simulink model "flexpes_phctrlr_sys"  (R2025b)
settings: Solver=VariableStepAuto  StartTime=0.0  StopTime=1e-6  RelTol=1e-3
values from neighbouring files (symbols this model uses):
  debouncer_cycles = 5    [choPLL_loop_impl.m]
  F_lock_thr = 1    [choPLL_loop_impl.m]
  FPGA_CLK = 125e6    (= 125000000)    [choPLL_loop_impl.m]
  FPGA_Ts = 1./FPGA_CLK    (= 8e-09)    [choPLL_loop_impl.m]
  IIR_C_X = G_loopfilt*my_num_loop_filtZ(1)    [choPLL_loop_impl.m]
  IIR_C_X1 = G_loopfilt*my_num_loop_filtZ(2)    [choPLL_loop_impl.m]
  IIR_C_Y1 = -my_den_loop_filtZ(2)    [choPLL_loop_impl.m]
  max_unwrap_periods = 50    [choPLL_loop_impl.m]
  PFD_CLK = 100e3    (= 100000)    [choPLL_loop_impl.m]
  PFD_Ts = 1./PFD_CLK    (= 1e-05)    [choPLL_loop_impl.m]
  PH_lock_thr = 4    [choPLL_loop_impl.m]
  PHCTRLR_CLK = 100    [choPLL_loop_impl.m]
  PHCTRLR_Ts = 1./PHCTRLR_CLK    (= 0.01)    [choPLL_loop_impl.m]
  TDC_cnt_per_period = round(FPGA_CLK/Fref)    [choPLL_loop_impl.m]
  unwrap_res_period_thr = 0    [choPLL_loop_impl.m]
  unwrap_reset_inhibit_cycles = 20000    [choPLL_loop_impl.m]
  wrap_detect_thr = round(TDC_cnt_per_period*0.55)    [choPLL_loop_impl.m]
libraries: hdlBasic x276, hdlUtilities x4, hdlDSPIP x4, vmcUtilities x1
(part 2 of 3)

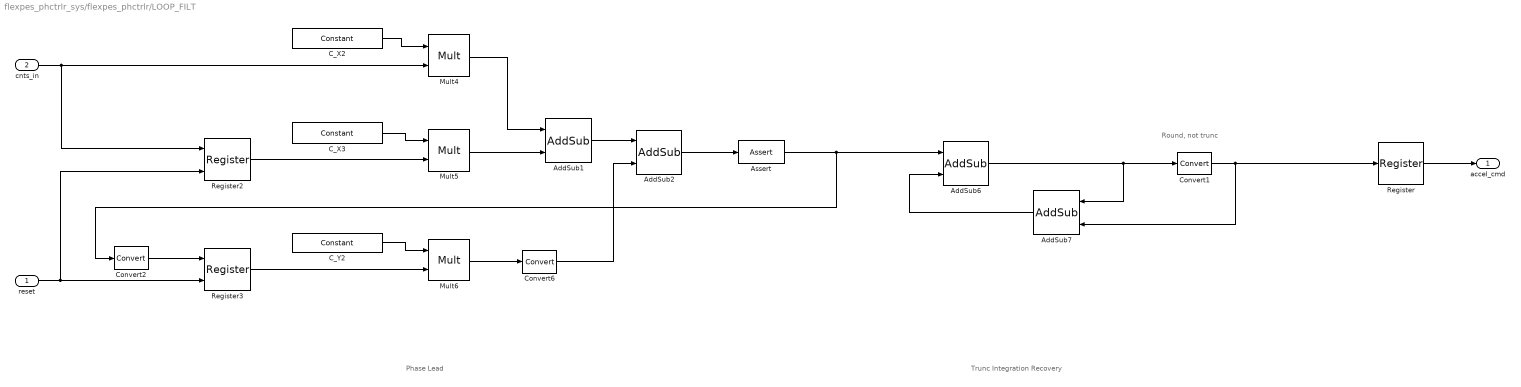
== system flexpes_phctrlr_sys/flexpes_phctrlr/LOOP_FILT ==
  note: Round, not trunc
  note: Phase Lead
  note: Trunc Integration Recovery
  reset : Inport
  cnts_in : Inport  Port=2
  AddSub1 : hdlBasic/AddSub  mode=Addition  use_carryin=off  use_carryout=off  en=off  latency=0  precision=Full  arith_type=Unsigned  n_bits=16  bin_pt=14  quantization=Truncate  overflow=Wrap  use_behavioral_HDL=off  hw_selection=Fabric  pipelined=off  XmcBlockStatus=1  maskContainerNames=tabcontainer1  block_type=addsub  block_config=sysgen:Addsub_config
  AddSub2 : hdlBasic/AddSub  mode=Addition  use_carryin=off  use_carryout=off  en=off  latency=0  precision=Full  arith_type=Unsigned  n_bits=16  bin_pt=14  quantization=Truncate  overflow=Wrap  use_behavioral_HDL=off  hw_selection=Fabric  pipelined=off  XmcBlockStatus=1  maskContainerNames=tabcontainer1  block_type=addsub  block_config=sysgen:Addsub_config
  AddSub6 : hdlBasic/AddSub  mode=Addition  use_carryin=off  use_carryout=off  en=off  latency=0  precision=User Defined  arith_type="Signed  (2's comp)"  n_bits=44  bin_pt=24  quantization="Round  (unbiased: +/- Inf)"  overflow=Saturate  use_behavioral_HDL=off  hw_selection=Fabric  pipelined=off  XmcBlockStatus=1  maskContainerNames=tabcontainer1  block_type=addsub  block_config=sysgen:Addsub_config
  AddSub7 : hdlBasic/AddSub  mode=Subtraction  use_carryin=off  use_carryout=off  en=off  latency=1  precision=User Defined  arith_type="Signed  (2's comp)"  n_bits=44  bin_pt=24  quantization="Round  (unbiased: +/- Inf)"  overflow=Saturate  use_behavioral_HDL=off  hw_selection=Fabric  pipelined=off  XmcBlockStatus=1  maskContainerNames=tabcontainer1  block_type=addsub  block_config=sysgen:Addsub_config
  Assert : hdlBasic/Assert  assert_type=off  type_source=Explicitly  gui_display_data_type=Fixed-point  arith_type=Signed (2's comp)  n_bits=16  bin_pt=14  preci_type=Single  exp_width=8  frac_width=24  assert_rate=on  rate_source=Explicitly  period=PHCTRLR_Ts  output_port=on  XmcBlockStatus=1  maskContainerNames=group1  block_type=assert  block_config=sysgen:assert_config  block_width=609  block_height=900
  C_X2 : hdlBasic/Constant  const=IIR_C_X  gui_display_data_type=Fixed-point  arith_type=Signed (2's comp)  n_bits=18  bin_pt=17  preci_type=Single  exp_width=8  frac_width=24  explicit_period=on  period=PHCTRLR_Ts  XmcBlockStatus=1  maskContainerNames=tabcontainer1  block_type=constant  block_config=sysgen:Constant_config
  C_X3 : hdlBasic/Constant  const=IIR_C_X1  gui_display_data_type=Fixed-point  arith_type=Signed (2's comp)  n_bits=18  bin_pt=17  preci_type=Single  exp_width=8  frac_width=24  explicit_period=on  period=PHCTRLR_Ts  XmcBlockStatus=1  maskContainerNames=tabcontainer1  block_type=constant  block_config=sysgen:Constant_config
  C_Y2 : hdlBasic/Constant  const=IIR_C_Y1  gui_display_data_type=Fixed-point  arith_type=Signed (2's comp)  n_bits=18  bin_pt=17  preci_type=Single  exp_width=8  frac_width=24  explicit_period=on  period=PHCTRLR_Ts  XmcBlockStatus=1  maskContainerNames=tabcontainer1  block_type=constant  block_config=sysgen:Constant_config
  Convert1 : hdlBasic/Convert  gui_display_data_type=Fixed-point  arith_type=Signed (2's comp)  n_bits=22  bin_pt=0  float_type=Single  exp_bits=8  fraction_bits=24  quantization="Round  (unbiased: Even Values)"  overflow=Saturate  en=off  latency=0  pipeline=off  XmcBlockStatus=1  maskContainerNames=group2  block_type=convert  block_config=sysgen:Convert_config  block_width=595  block_height=885
  Convert2 : hdlBasic/Convert  gui_display_data_type=Fixed-point  arith_type=Signed (2's comp)  n_bits=42  bin_pt=24  float_type=Single  exp_bits=8  fraction_bits=24  quantization="Round  (unbiased: Even Values)"  overflow=Saturate  en=off  latency=0  pipeline=off  XmcBlockStatus=1  maskContainerNames=group2  block_type=convert  block_config=sysgen:Convert_config  block_width=595  block_height=885
  Convert6 : hdlBasic/Convert  gui_display_data_type=Fixed-point  arith_type=Signed (2's comp)  n_bits=43  bin_pt=24  float_type=Single  exp_bits=8  fraction_bits=24  quantization="Round  (unbiased: Even Values)"  overflow=Saturate  en=off  latency=0  pipeline=off  XmcBlockStatus=1  maskContainerNames=group2  block_type=convert  block_config=sysgen:Convert_config  block_width=595  block_height=885
  Mult4 : hdlBasic/Mult  precision=Full  arith_type="Signed  (2's comp)"  n_bits=16  bin_pt=14  quantization=Truncate  overflow=Wrap  en=off  latency=0  opt_float=off  fp_mult_usage=No Usage  use_behavioral_HDL=off  opt=Speed  use_embedded=on  optimum_pipeline=off  pipeline=on  use_rpm=on  placement_style=Triangular  XmcBlockStatus=1  maskContainerNames=group1  block_type=mult  block_config=sysgen:Mult_config  block_width=598  block_height=876
  Mult5 : hdlBasic/Mult  precision=Full  arith_type="Signed  (2's comp)"  n_bits=16  bin_pt=14  quantization=Truncate  overflow=Wrap  en=off  latency=0  opt_float=off  fp_mult_usage=No Usage  use_behavioral_HDL=off  opt=Speed  use_embedded=on  optimum_pipeline=off  pipeline=on  use_rpm=on  placement_style=Triangular  XmcBlockStatus=1  maskContainerNames=group1  block_type=mult  block_config=sysgen:Mult_config  block_width=598  block_height=876
  Mult6 : hdlBasic/Mult  precision=Full  arith_type="Signed  (2's comp)"  n_bits=16  bin_pt=14  quantization=Truncate  overflow=Wrap  en=off  latency=0  opt_float=off  fp_mult_usage=No Usage  use_behavioral_HDL=off  opt=Speed  use_embedded=on  optimum_pipeline=off  pipeline=on  use_rpm=on  placement_style=Triangular  XmcBlockStatus=1  maskContainerNames=group1  block_type=mult  block_config=sysgen:Mult_config  block_width=598  block_height=876
  Register : hdlBasic/Register  init=0  rst=off  en=off  XmcBlockStatus=1  maskContainerNames=tabcontainer1  block_type=register  block_config=sysgen:Register_config
  Register2 : hdlBasic/Register  init=0  rst=on  en=off  XmcBlockStatus=1  maskContainerNames=tabcontainer1  block_type=register  block_config=sysgen:Register_config
  Register3 : hdlBasic/Register  init=0  rst=on  en=off  XmcBlockStatus=1  maskContainerNames=tabcontainer1  block_type=register  block_config=sysgen:Register_config
  accel_cmd : Outport
  wires:
  reset/1 -> Register2/2, Register3/2
  Convert6/1 -> AddSub2/2
  Mult4/1 -> AddSub1/1
  C_X3/1 -> Mult5/1
  Convert2/1 -> Register3/1
  Mult5/1 -> AddSub1/2
  C_X2/1 -> Mult4/1
  Mult6/1 -> Convert6/1
  cnts_in/1 -> Mult4/2, Register2/1
  Register2/1 -> Mult5/2
  C_Y2/1 -> Mult6/1
  AddSub2/1 -> Assert/1
  AddSub1/1 -> AddSub2/1
  Register3/1 -> Mult6/2
  Register/1 -> accel_cmd/1
  AddSub6/1 -> AddSub7/1, Convert1/1
  Convert1/1 -> Register/1, AddSub7/2
  AddSub7/1 -> AddSub6/2
  Assert/1 -> Convert2/1, AddSub6/1

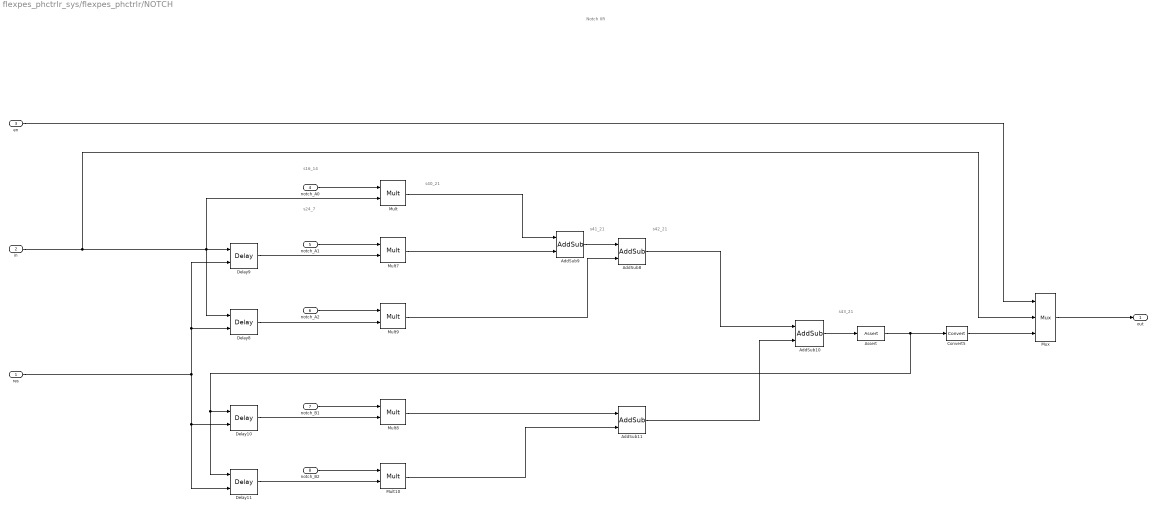
== system flexpes_phctrlr_sys/flexpes_phctrlr/NOTCH ==
  note: s16_14
  note: Notch IIR
  note: s24_7
  note: s40_21
  note: s42_21
  note: s43_21
  note: s41_21
  res : Inport
  in : Inport  Port=2
  en : Inport  Port=3
  notch_A0 : Inport  Port=4  OutDataTypeStr=fixdt(1,16,14)
  notch_A1 : Inport  Port=5  OutDataTypeStr=fixdt(1,16,14)
  notch_A2 : Inport  Port=6  OutDataTypeStr=fixdt(1,16,14)
  notch_B1 : Inport  Port=7  OutDataTypeStr=fixdt(1,16,14)
  notch_B2 : Inport  Port=8  OutDataTypeStr=fixdt(1,16,14)
  AddSub10 : hdlBasic/AddSub  mode=Subtraction  use_carryin=off  use_carryout=off  en=off  latency=0  precision=Full  arith_type="Signed  (2's comp)"  n_bits=62  bin_pt=40  quantization="Round  (unbiased: +/- Inf)"  overflow=Saturate  use_behavioral_HDL=off  hw_selection=Fabric  pipelined=off  XmcBlockStatus=1  maskContainerNames=tabcontainer1  block_type=addsub  block_config=sysgen:Addsub_config
  AddSub11 : hdlBasic/AddSub  mode=Addition  use_carryin=off  use_carryout=off  en=off  latency=0  precision=Full  arith_type="Signed  (2's comp)"  n_bits=62  bin_pt=40  quantization="Round  (unbiased: +/- Inf)"  overflow=Saturate  use_behavioral_HDL=off  hw_selection=Fabric  pipelined=off  XmcBlockStatus=1  maskContainerNames=tabcontainer1  block_type=addsub  block_config=sysgen:Addsub_config
  AddSub8 : hdlBasic/AddSub  mode=Addition  use_carryin=off  use_carryout=off  en=off  latency=0  precision=Full  arith_type=Unsigned  n_bits=16  bin_pt=14  quantization=Truncate  overflow=Wrap  use_behavioral_HDL=off  hw_selection=Fabric  pipelined=off  XmcBlockStatus=1  maskContainerNames=tabcontainer1  block_type=addsub  block_config=sysgen:Addsub_config
  AddSub9 : hdlBasic/AddSub  mode=Addition  use_carryin=off  use_carryout=off  en=off  latency=0  precision=Full  arith_type=Unsigned  n_bits=16  bin_pt=14  quantization=Truncate  overflow=Wrap  use_behavioral_HDL=off  hw_selection=Fabric  pipelined=off  XmcBlockStatus=1  maskContainerNames=tabcontainer1  block_type=addsub  block_config=sysgen:Addsub_config
  Assert : hdlBasic/Assert  assert_type=off  type_source=Explicitly  gui_display_data_type=Fixed-point  arith_type=Signed (2's comp)  n_bits=16  bin_pt=14  preci_type=Single  exp_width=8  frac_width=24  assert_rate=on  rate_source=Explicitly  period=PHCTRLR_Ts  output_port=on  XmcBlockStatus=1  maskContainerNames=group1  block_type=assert  block_config=sysgen:assert_config  block_width=609  block_height=900
  Convert5 : hdlBasic/Convert  gui_display_data_type=Fixed-point  arith_type=Signed (2's comp)  n_bits=24  bin_pt=7  float_type=Single  exp_bits=8  fraction_bits=24  quantization="Round  (unbiased: Even Values)"  overflow=Saturate  en=off  latency=1  pipeline=off  XmcBlockStatus=1  maskContainerNames=group2  block_type=convert  block_config=sysgen:Convert_config  block_width=595  block_height=885
  Delay10 : hdlBasic/Delay  rst=on  en=off  latency=1  reg_retiming=off  XmcBlockStatus=1  maskContainerNames=group1  block_type=delay  block_config=sysgen:Delay_config
  Delay11 : hdlBasic/Delay  rst=on  en=off  latency=2  reg_retiming=off  XmcBlockStatus=1  maskContainerNames=group1  block_type=delay  block_config=sysgen:Delay_config
  Delay8 : hdlBasic/Delay  rst=on  en=off  latency=2  reg_retiming=off  XmcBlockStatus=1  maskContainerNames=group1  block_type=delay  block_config=sysgen:Delay_config
  Delay9 : hdlBasic/Delay  rst=on  en=off  latency=1  reg_retiming=off  XmcBlockStatus=1  maskContainerNames=group1  block_type=delay  block_config=sysgen:Delay_config
  Mult : hdlBasic/Mult  precision=Full  arith_type="Signed  (2's comp)"  n_bits=16  bin_pt=14  quantization=Truncate  overflow=Wrap  en=off  latency=0  opt_float=off  fp_mult_usage=No Usage  use_behavioral_HDL=off  opt=Speed  use_embedded=on  optimum_pipeline=off  pipeline=on  use_rpm=on  placement_style=Triangular  XmcBlockStatus=1  maskContainerNames=group1  block_type=mult  block_config=sysgen:Mult_config  block_width=598  block_height=876
  Mult10 : hdlBasic/Mult  precision=User Defined  arith_type="Signed  (2's comp)"  n_bits=41  bin_pt=21  quantization="Round  (unbiased: +/- Inf)"  overflow=Saturate  en=off  latency=0  opt_float=off  fp_mult_usage=No Usage  use_behavioral_HDL=off  opt=Speed  use_embedded=on  optimum_pipeline=off  pipeline=on  use_rpm=on  placement_style=Triangular  XmcBlockStatus=1  maskContainerNames=group1  block_type=mult  block_config=sysgen:Mult_config  block_width=598  block_height=876
  Mult7 : hdlBasic/Mult  precision=Full  arith_type="Signed  (2's comp)"  n_bits=16  bin_pt=14  quantization=Truncate  overflow=Wrap  en=off  latency=0  opt_float=off  fp_mult_usage=No Usage  use_behavioral_HDL=off  opt=Speed  use_embedded=on  optimum_pipeline=off  pipeline=on  use_rpm=on  placement_style=Triangular  XmcBlockStatus=1  maskContainerNames=group1  block_type=mult  block_config=sysgen:Mult_config  block_width=598  block_height=876
  Mult8 : hdlBasic/Mult  precision=User Defined  arith_type="Signed  (2's comp)"  n_bits=41  bin_pt=21  quantization="Round  (unbiased: +/- Inf)"  overflow=Saturate  en=off  latency=0  opt_float=off  fp_mult_usage=No Usage  use_behavioral_HDL=off  opt=Speed  use_embedded=on  optimum_pipeline=off  pipeline=on  use_rpm=on  placement_style=Triangular  XmcBlockStatus=1  maskContainerNames=group1  block_type=mult  block_config=sysgen:Mult_config  block_width=598  block_height=876
  Mult9 : hdlBasic/Mult  precision=Full  arith_type="Signed  (2's comp)"  n_bits=16  bin_pt=14  quantization=Truncate  overflow=Wrap  en=off  latency=0  opt_float=off  fp_mult_usage=No Usage  use_behavioral_HDL=off  opt=Speed  use_embedded=on  optimum_pipeline=off  pipeline=on  use_rpm=on  placement_style=Triangular  XmcBlockStatus=1  maskContainerNames=group1  block_type=mult  block_config=sysgen:Mult_config  block_width=598  block_height=876
  Mux : hdlBasic/Mux  inputs=2  en=off  latency=1  precision=Full  arith_type=Unsigned  n_bits=16  bin_pt=14  quantization=Truncate  overflow=Wrap  XmcBlockStatus=1  maskContainerNames=tabcontainer1  block_type=mux  block_config=sysgen:Mux_config
  out : Outport
  wires:
  AddSub11/1 -> AddSub10/2
  Mult7/1 -> AddSub9/2
  notch_A1/1 -> Mult7/1
  Mult9/1 -> AddSub8/2
  Delay9/1 -> Mult7/2
  in/1 -> Mux/2, Mult/2, Delay8/1, Delay9/1
  notch_B1/1 -> Mult8/1
  AddSub8/1 -> AddSub10/1
  Convert5/1 -> Mux/3
  AddSub10/1 -> Assert/1
  notch_A2/1 -> Mult9/1
  Delay8/1 -> Mult9/2
  notch_A0/1 -> Mult/1
  Mult10/1 -> AddSub11/2
  Mult8/1 -> AddSub11/1
  Delay10/1 -> Mult8/2
  Delay11/1 -> Mult10/2
  AddSub9/1 -> AddSub8/1
  en/1 -> Mux/1
  Mult/1 -> AddSub9/1
  res/1 -> Delay11/2, Delay10/2, Delay9/2, Delay8/2
  Mux/1 -> out/1
  notch_B2/1 -> Mult10/1
  Assert/1 -> Delay11/1, Delay10/1, Convert5/1

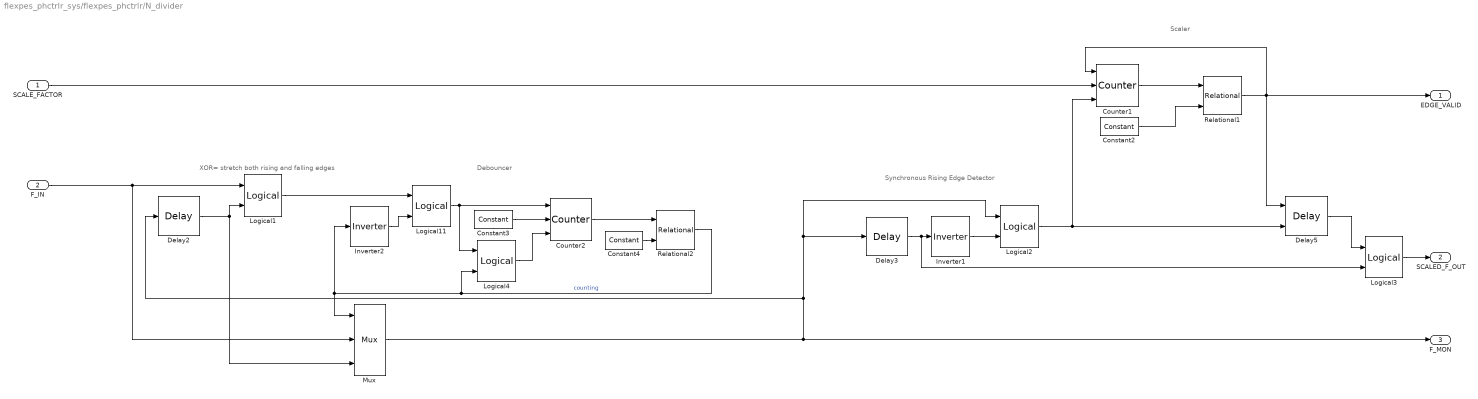
== system flexpes_phctrlr_sys/flexpes_phctrlr/N_divider ==
  note: XOR= stretch both rising and falling edges
  note: Debouncer
  note: Scaler
  note: Synchronous Rising Edge Detector
  SCALE_FACTOR : Inport
  F_IN : Inport  Port=2
  Constant2 : hdlBasic/Constant  const=1.0  gui_display_data_type=Fixed-point  arith_type=Unsigned  n_bits=16  bin_pt=0  preci_type=Single  exp_width=8  frac_width=24  explicit_period=off  period=1  XmcBlockStatus=1  maskContainerNames=tabcontainer1  block_type=constant  block_config=sysgen:Constant_config
  Constant3 : hdlBasic/Constant  const=debouncer_cycles  gui_display_data_type=Fixed-point  arith_type=Unsigned  n_bits=7  bin_pt=0  preci_type=Single  exp_width=8  frac_width=24  explicit_period=off  period=1  XmcBlockStatus=1  maskContainerNames=tabcontainer1  block_type=constant  block_config=sysgen:Constant_config
  Constant4 : hdlBasic/Constant  const=1  gui_display_data_type=Fixed-point  arith_type=Unsigned  n_bits=7  bin_pt=0  preci_type=Single  exp_width=8  frac_width=24  explicit_period=off  period=1  XmcBlockStatus=1  maskContainerNames=tabcontainer1  block_type=constant  block_config=sysgen:Constant_config
  Counter1 : hdlBasic/Counter  cnt_type=Free running  cnt_to=2  operation=Down  start_count=1  cnt_by_val=1  arith_type=Unsigned  n_bits=16  bin_pt=0  load_pin=on  rst=off  en=on  explicit_period=Explicit  period=FPGA_Ts  use_behavioral_HDL=off  implementation=Fabric  XmcBlockStatus=1  maskContainerNames=group1  block_type=counter  block_config=sysgen:Counter_config  block_width=531  block_height=1023
  Counter2 : hdlBasic/Counter  cnt_type=Free running  cnt_to=2  operation=Down  start_count=1  cnt_by_val=1  arith_type=Unsigned  n_bits=7  bin_pt=0  load_pin=on  rst=off  en=on  explicit_period=Explicit  period=FPGA_Ts  use_behavioral_HDL=off  implementation=Fabric  XmcBlockStatus=1  maskContainerNames=group1  block_type=counter  block_config=sysgen:Counter_config  block_width=531  block_height=1023
  Delay2 : hdlBasic/Delay  rst=off  en=off  latency=1  reg_retiming=off  XmcBlockStatus=1  maskContainerNames=group1  block_type=delay  block_config=sysgen:Delay_config
  Delay3 : hdlBasic/Delay  rst=off  en=off  latency=1  reg_retiming=off  XmcBlockStatus=1  maskContainerNames=group1  block_type=delay  block_config=sysgen:Delay_config
  Delay5 : hdlBasic/Delay  rst=off  en=on  latency=1  reg_retiming=off  XmcBlockStatus=1  maskContainerNames=group1  block_type=delay  block_config=sysgen:Delay_config
  Inverter1 : hdlBasic/Inverter  en=off  latency=0  XmcBlockStatus=1  maskContainerNames=group2  block_type=inv  block_config=sysgen:Inverter_config
  Inverter2 : hdlBasic/Inverter  en=off  latency=0  XmcBlockStatus=1  maskContainerNames=group2  block_type=inv  block_config=sysgen:Inverter_config
  Logical1 : hdlBasic/Logical  logical_function=XOR  inputs=2  en=off  latency=0  precision=Full  arith_type=Unsigned  n_bits=16  bin_pt=0  align_bp=on  overflow=[]  quantization=[]  XmcBlockStatus=1  maskContainerNames=tabcontainer1  block_type=logical  block_config=sysgen:Logical_config
  Logical11 : hdlBasic/Logical  logical_function=AND  inputs=2  en=off  latency=0  precision=Full  arith_type=Unsigned  n_bits=16  bin_pt=0  align_bp=on  overflow=[]  quantization=[]  XmcBlockStatus=1  maskContainerNames=tabcontainer1  block_type=logical  block_config=sysgen:Logical_config
  Logical2 : hdlBasic/Logical  logical_function=AND  inputs=2  en=off  latency=0  precision=Full  arith_type=Unsigned  n_bits=16  bin_pt=0  align_bp=on  overflow=[]  quantization=[]  XmcBlockStatus=1  maskContainerNames=tabcontainer1  block_type=logical  block_config=sysgen:Logical_config
  Logical3 : hdlBasic/Logical  logical_function=AND  inputs=2  en=off  latency=0  precision=Full  arith_type=Unsigned  n_bits=16  bin_pt=0  align_bp=on  overflow=[]  quantization=[]  XmcBlockStatus=1  maskContainerNames=tabcontainer1  block_type=logical  block_config=sysgen:Logical_config
  Logical4 : hdlBasic/Logical  logical_function=OR  inputs=2  en=off  latency=0  precision=Full  arith_type=Unsigned  n_bits=16  bin_pt=0  align_bp=on  overflow=[]  quantization=[]  XmcBlockStatus=1  maskContainerNames=tabcontainer1  block_type=logical  block_config=sysgen:Logical_config
  Mux : hdlBasic/Mux  inputs=2  en=off  latency=0  precision=Full  arith_type=Unsigned  n_bits=16  bin_pt=14  quantization=Truncate  overflow=Wrap  XmcBlockStatus=1  maskContainerNames=tabcontainer1  block_type=mux  block_config=sysgen:Mux_config
  Relational1 : hdlBasic/Relational  mode=a=b  op_type=Bool  en=off  latency=0  XmcBlockStatus=1  maskContainerNames=tabcontainer1  block_type=relational  block_config=sysgen:Relational_config
  Relational2 : hdlBasic/Relational  mode=a!=b  op_type=Bool  en=off  latency=0  XmcBlockStatus=1  maskContainerNames=tabcontainer1  block_type=relational  block_config=sysgen:Relational_config
  EDGE_VALID : Outport
  SCALED_F_OUT : Outport  Port=2
  F_MON : Outport  Port=3
  wires:
  Delay2/1 -> Logical1/2, Mux/3
  Logical2/1 -> Delay5/2, Counter1/3
  Constant4/1 -> Relational2/2
  Inverter2/1 -> Logical11/2
  Counter2/1 -> Relational2/1
  Constant3/1 -> Counter2/2
  Relational2/1 -> Mux/1, Inverter2/1, Logical4/2  "counting"
  Delay5/1 -> Logical3/1
  Delay3/1 -> Inverter1/1, Logical3/2
  F_IN/1 -> Logical1/1, Mux/2
  Counter1/1 -> Relational1/1
  Inverter1/1 -> Logical2/2
  Constant2/1 -> Relational1/2
  SCALE_FACTOR/1 -> Counter1/2
  Logical11/1 -> Logical4/1, Counter2/1
  Logical3/1 -> SCALED_F_OUT/1
  Logical4/1 -> Counter2/3
  Logical1/1 -> Logical11/1
  Relational1/1 -> EDGE_VALID/1, Delay5/1, Counter1/1
  Mux/1 -> F_MON/1, Delay2/1, Logical2/1, Delay3/1

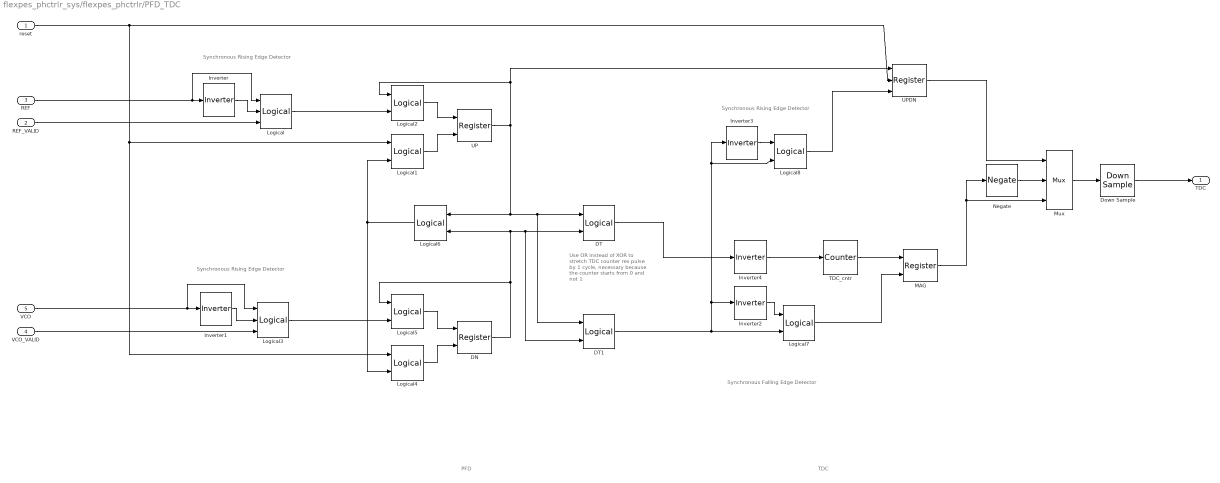
== system flexpes_phctrlr_sys/flexpes_phctrlr/PFD_TDC ==
  note: Synchronous Rising Edge Detector
  note: Synchronous Rising Edge Detector
  note: Synchronous Rising Edge Detector
  note: Synchronous Falling Edge Detector
  note: PFD
  note: TDC
  note: Use OR instead of XOR to
      | stretch TDC counter res
      | pulse by 1 cycle, necessary
      | because the counter starts
      | from 0 and not 1
  reset : Inport  SampleTime=FPGA_Ts
  REF_VALID : Inport  Port=2  SampleTime=FPGA_Ts
  REF : Inport  Port=3  SampleTime=FPGA_Ts
  VCO_VALID : Inport  Port=4  SampleTime=FPGA_Ts
  VCO : Inport  Port=5  SampleTime=FPGA_Ts
  DN : hdlBasic/Register  init=0  rst=on  en=off  XmcBlockStatus=1  maskContainerNames=tabcontainer1  block_type=register  block_config=sysgen:Register_config
  DT : hdlBasic/Logical  logical_function=OR  inputs=2  en=off  latency=0  precision=Full  arith_type=Unsigned  n_bits=16  bin_pt=0  align_bp=on  overflow=[]  quantization=[]  XmcBlockStatus=1  maskContainerNames=tabcontainer1  block_type=logical  block_config=sysgen:Logical_config
  DT1 : hdlBasic/Logical  logical_function=XOR  inputs=2  en=off  latency=0  precision=Full  arith_type=Unsigned  n_bits=16  bin_pt=0  align_bp=on  overflow=[]  quantization=[]  XmcBlockStatus=1  maskContainerNames=tabcontainer1  block_type=logical  block_config=sysgen:Logical_config
  Down Sample : hdlBasic/Down Sample  sample_ratio=FPGA_CLK/PFD_CLK  sample_phase="Last Value of Frame  (most efficient)"  en=off  rst=off  latency=1  XmcBlockStatus=1  maskContainerNames=group1  block_type=dsamp  block_config=sysgen:Downsample_config
  Inverter{,1..3} (4 alike) : hdlBasic/Inverter  en=off  latency=1  XmcBlockStatus=1  maskContainerNames=group2  block_type=inv  block_config=sysgen:Inverter_config
  Inverter4 : hdlBasic/Inverter  en=off  latency=0  XmcBlockStatus=1  maskContainerNames=group2  block_type=inv  block_config=sysgen:Inverter_config
  Logical : hdlBasic/Logical  logical_function=AND  inputs=3  en=off  latency=0  precision=Full  arith_type=Unsigned  n_bits=16  bin_pt=0  align_bp=on  overflow=[]  quantization=[]  XmcBlockStatus=1  maskContainerNames=tabcontainer1  block_type=logical  block_config=sysgen:Logical_config
  Logical{1..2,4..5} (4 alike) : hdlBasic/Logical  logical_function=OR  inputs=2  en=off  latency=0  precision=Full  arith_type=Unsigned  n_bits=16  bin_pt=0  align_bp=on  overflow=[]  quantization=[]  XmcBlockStatus=1  maskContainerNames=tabcontainer1  block_type=logical  block_config=sysgen:Logical_config
  Logical3 : hdlBasic/Logical  logical_function=AND  inputs=3  en=off  latency=0  precision=Full  arith_type=Unsigned  n_bits=16  bin_pt=0  align_bp=on  overflow=[]  quantization=[]  XmcBlockStatus=1  maskContainerNames=tabcontainer1  block_type=logical  block_config=sysgen:Logical_config
  Logical6 : hdlBasic/Logical  logical_function=AND  inputs=2  en=off  latency=1  precision=Full  arith_type=Unsigned  n_bits=16  bin_pt=0  align_bp=on  overflow=[]  quantization=[]  XmcBlockStatus=1  maskContainerNames=tabcontainer1  block_type=logical  block_config=sysgen:Logical_config
  Logical7 : hdlBasic/Logical  logical_function=NOR  inputs=2  en=off  latency=0  precision=Full  arith_type=Unsigned  n_bits=16  bin_pt=0  align_bp=on  overflow=[]  quantization=[]  XmcBlockStatus=1  maskContainerNames=tabcontainer1  block_type=logical  block_config=sysgen:Logical_config
  Logical8 : hdlBasic/Logical  logical_function=AND  inputs=2  en=off  latency=0  precision=Full  arith_type=Unsigned  n_bits=16  bin_pt=0  align_bp=on  overflow=[]  quantization=[]  XmcBlockStatus=1  maskContainerNames=tabcontainer1  block_type=logical  block_config=sysgen:Logical_config
  MAG : hdlBasic/Register  init=0  rst=off  en=on  XmcBlockStatus=1  maskContainerNames=tabcontainer1  block_type=register  block_config=sysgen:Register_config
  Mux : hdlBasic/Mux  inputs=2  en=off  latency=1  precision=Full  arith_type=Unsigned  n_bits=16  bin_pt=14  quantization=Truncate  overflow=Wrap  XmcBlockStatus=1  maskContainerNames=tabcontainer1  block_type=mux  block_config=sysgen:Mux_config
  Negate : hdlBasic/Negate  precision=User Defined  arith_type="Signed  (2's comp)"  n_bits=17  bin_pt=0  quantization=Truncate  overflow=Wrap  en=off  latency=0  XmcBlockStatus=1  maskContainerNames=tabcontainer1  block_type=negate  block_config=sysgen:Negate_config
  TDC_cntr : hdlBasic/Counter  cnt_type=Free running  cnt_to=Inf  operation=Up  start_count=0  cnt_by_val=1  arith_type="Signed  (2's comp)"  n_bits=17  bin_pt=0  load_pin=off  rst=on  en=off  explicit_period=Explicit  period=FPGA_Ts  use_behavioral_HDL=off  implementation=DSP48  XmcBlockStatus=1  maskContainerNames=group1  block_type=counter  block_config=sysgen:Counter_config  block_width=531  block_height=1023
  UP : hdlBasic/Register  init=0  rst=on  en=off  XmcBlockStatus=1  maskContainerNames=tabcontainer1  block_type=register  block_config=sysgen:Register_config
  UPDN : hdlBasic/Register  init=0  rst=on  en=on  XmcBlockStatus=1  maskContainerNames=tabcontainer1  block_type=register  block_config=sysgen:Register_config
  TDC : Outport  SampleTime=PFD_Ts
  wires:
  Logical3/1 -> Logical5/2
  VCO/1 -> Logical3/1, Inverter1/1
  reset/1 -> Logical4/1, Logical1/1, UPDN/2
  Logical5/1 -> DN/1
  Logical2/1 -> UP/1
  DN/1 -> Logical5/1, Logical6/2, DT1/2, DT/2
  REF/1 -> Logical/1, Inverter/1
  DT/1 -> Inverter4/1
  Logical4/1 -> DN/2
  MAG/1 -> Negate/1, Mux/3
  Down Sample/1 -> TDC/1
  Inverter3/1 -> Logical8/1
  Logical8/1 -> UPDN/3
  UP/1 -> UPDN/1, Logical2/1, DT1/1, DT/1, Logical6/1
  Logical6/1 -> Logical1/2, Logical4/2
  Logical1/1 -> UP/2
  UPDN/1 -> Mux/1
  Mux/1 -> Down Sample/1
  Logical/1 -> Logical2/2
  Negate/1 -> Mux/2
  Logical7/1 -> MAG/2
  Inverter2/1 -> Logical7/1
  TDC_cntr/1 -> MAG/1
  Inverter4/1 -> TDC_cntr/1
  DT1/1 -> Logical8/2, Inverter3/1, Inverter2/1, Logical7/2
  REF_VALID/1 -> Logical/3
  Inverter1/1 -> Logical3/2
  VCO_VALID/1 -> Logical3/3
  Inverter/1 -> Logical/2

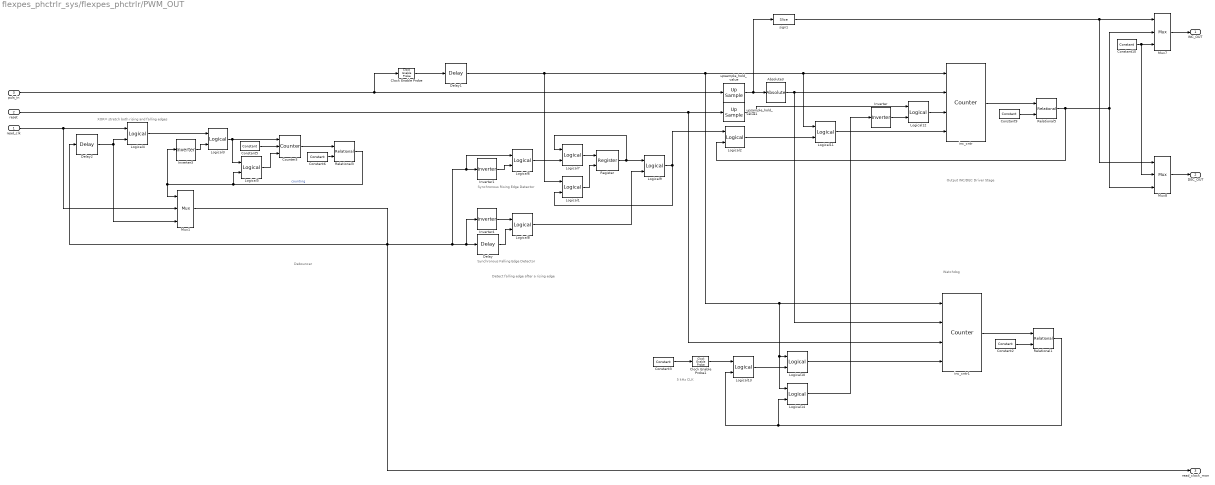
== system flexpes_phctrlr_sys/flexpes_phctrlr/PWM_OUT ==
  note: Output INC/DEC Driver Stage
  note: XOR= stretch both rising and falling edges
  note: Synchronous Rising Edge Detector
  note: Detect falling edge after a rising edge
  note: Debouncer
  note: Watchdog
  note: Synchronous Falling Edge Detector
  note: 5 kHz CLK
  read_clk : Inport
  reset : Inport  Port=2
  puls_in : Inport  Port=3
  Absolute3 : hdlBasic/Absolute  precision=User Defined  arith_type="Signed  (2's comp)"  n_bits=22  bin_pt=0  quantization=Truncate  overflow=Wrap  en=off  latency=0  XmcBlockStatus=1  maskContainerNames=tabcontainer1  block_type=abs  block_config=sysgen:Abs_config
  Clock Enable Probe : hdlUtilities/Clock Enable Probe  inherit_constraints=on  XmcBlockStatus=1  maskContainerNames=group1  block_type=ceprobe  block_config=sysgen:CEProbe_config
  Clock Enable Probe1 : hdlUtilities/Clock Enable Probe  inherit_constraints=on  XmcBlockStatus=1  maskContainerNames=group1  block_type=ceprobe  block_config=sysgen:CEProbe_config
  Constant10 : hdlBasic/Constant  const=0  gui_display_data_type=Boolean  arith_type=Boolean  n_bits=22  bin_pt=0  preci_type=Single  exp_width=8  frac_width=24  explicit_period=off  period=1  XmcBlockStatus=1  maskContainerNames=tabcontainer1  block_type=constant  block_config=sysgen:Constant_config
  Constant2 : hdlBasic/Constant  const=0  gui_display_data_type=Fixed-point  arith_type=Signed (2's comp)  n_bits=22  bin_pt=0  preci_type=Single  exp_width=8  frac_width=24  explicit_period=off  period=1  XmcBlockStatus=1  maskContainerNames=tabcontainer1  block_type=constant  block_config=sysgen:Constant_config
  Constant3 : hdlBasic/Constant  const=1  gui_display_data_type=Boolean  arith_type=Boolean  n_bits=7  bin_pt=0  preci_type=Single  exp_width=8  frac_width=24  explicit_period=on  period=PWM_Ts  XmcBlockStatus=1  maskContainerNames=tabcontainer1  block_type=constant  block_config=sysgen:Constant_config
  Constant5 : hdlBasic/Constant  const=debouncer_cycles  gui_display_data_type=Fixed-point  arith_type=Unsigned  n_bits=7  bin_pt=0  preci_type=Single  exp_width=8  frac_width=24  explicit_period=off  period=1  XmcBlockStatus=1  maskContainerNames=tabcontainer1  block_type=constant  block_config=sysgen:Constant_config
  Constant6 : hdlBasic/Constant  const=1  gui_display_data_type=Fixed-point  arith_type=Unsigned  n_bits=7  bin_pt=0  preci_type=Single  exp_width=8  frac_width=24  explicit_period=off  period=1  XmcBlockStatus=1  maskContainerNames=tabcontainer1  block_type=constant  block_config=sysgen:Constant_config
  Constant9 : hdlBasic/Constant  const=0  gui_display_data_type=Fixed-point  arith_type=Signed (2's comp)  n_bits=22  bin_pt=0  preci_type=Single  exp_width=8  frac_width=24  explicit_period=off  period=1  XmcBlockStatus=1  maskContainerNames=tabcontainer1  block_type=constant  block_config=sysgen:Constant_config
  Counter3 : hdlBasic/Counter  cnt_type=Free running  cnt_to=2  operation=Down  start_count=1  cnt_by_val=1  arith_type=Unsigned  n_bits=7  bin_pt=0  load_pin=on  rst=off  en=on  explicit_period=Explicit  period=FPGA_Ts  use_behavioral_HDL=off  implementation=Fabric  XmcBlockStatus=1  maskContainerNames=group1  block_type=counter  block_config=sysgen:Counter_config  block_width=531  block_height=1023
  Delay : hdlBasic/Delay  rst=off  en=off  latency=1  reg_retiming=off  XmcBlockStatus=1  maskContainerNames=group1  block_type=delay  block_config=sysgen:Delay_config
  Delay1 : hdlBasic/Delay  rst=off  en=off  latency=1  reg_retiming=off  XmcBlockStatus=1  maskContainerNames=group1  block_type=delay  block_config=sysgen:Delay_config
  Delay2 : hdlBasic/Delay  rst=off  en=off  latency=1  reg_retiming=off  XmcBlockStatus=1  maskContainerNames=group1  block_type=delay  block_config=sysgen:Delay_config
  Inverter : hdlBasic/Inverter  en=off  latency=0  XmcBlockStatus=1  maskContainerNames=group2  block_type=inv  block_config=sysgen:Inverter_config
  Inverter1 : hdlBasic/Inverter  en=off  latency=1  XmcBlockStatus=1  maskContainerNames=group2  block_type=inv  block_config=sysgen:Inverter_config
  Inverter3 : hdlBasic/Inverter  en=off  latency=0  XmcBlockStatus=1  maskContainerNames=group2  block_type=inv  block_config=sysgen:Inverter_config
  Inverter4 : hdlBasic/Inverter  en=off  latency=0  XmcBlockStatus=1  maskContainerNames=group2  block_type=inv  block_config=sysgen:Inverter_config
  Logical{1,5,7,10..12,14} (7 alike) : hdlBasic/Logical  logical_function=OR  inputs=2  en=off  latency=0  precision=Full  arith_type=Unsigned  n_bits=16  bin_pt=0  align_bp=on  overflow=[]  quantization=[]  XmcBlockStatus=1  maskContainerNames=tabcontainer1  block_type=logical  block_config=sysgen:Logical_config
  Logical{2..3,6,8..9,13} (6 alike) : hdlBasic/Logical  logical_function=AND  inputs=2  en=off  latency=0  precision=Full  arith_type=Unsigned  n_bits=16  bin_pt=0  align_bp=on  overflow=[]  quantization=[]  XmcBlockStatus=1  maskContainerNames=tabcontainer1  block_type=logical  block_config=sysgen:Logical_config
  Logical4 : hdlBasic/Logical  logical_function=XOR  inputs=2  en=off  latency=0  precision=Full  arith_type=Unsigned  n_bits=16  bin_pt=0  align_bp=on  overflow=[]  quantization=[]  XmcBlockStatus=1  maskContainerNames=tabcontainer1  block_type=logical  block_config=sysgen:Logical_config
  Mux1 : hdlBasic/Mux  inputs=2  en=off  latency=0  precision=Full  arith_type=Unsigned  n_bits=16  bin_pt=14  quantization=Truncate  overflow=Wrap  XmcBlockStatus=1  maskContainerNames=tabcontainer1  block_type=mux  block_config=sysgen:Mux_config
  Mux7 : hdlBasic/Mux  inputs=2  en=off  latency=0  precision=Full  arith_type=Unsigned  n_bits=16  bin_pt=14  quantization=Truncate  overflow=Wrap  XmcBlockStatus=1  maskContainerNames=tabcontainer1  block_type=mux  block_config=sysgen:Mux_config
  Mux8 : hdlBasic/Mux  inputs=2  en=off  latency=0  precision=Full  arith_type=Unsigned  n_bits=16  bin_pt=14  quantization=Truncate  overflow=Wrap  XmcBlockStatus=1  maskContainerNames=tabcontainer1  block_type=mux  block_config=sysgen:Mux_config
  Register : hdlBasic/Register  init=0  rst=on  en=off  XmcBlockStatus=1  maskContainerNames=tabcontainer1  block_type=register  block_config=sysgen:Register_config
  Relational1 : hdlBasic/Relational  mode=a!=b  op_type=Bool  en=off  latency=0  XmcBlockStatus=1  maskContainerNames=tabcontainer1  block_type=relational  block_config=sysgen:Relational_config
  Relational3 : hdlBasic/Relational  mode=a!=b  op_type=Bool  en=off  latency=0  XmcBlockStatus=1  maskContainerNames=tabcontainer1  block_type=relational  block_config=sysgen:Relational_config
  Relational5 : hdlBasic/Relational  mode=a!=b  op_type=Bool  en=off  latency=0  XmcBlockStatus=1  maskContainerNames=tabcontainer1  block_type=relational  block_config=sysgen:Relational_config
  inc_cntr : hdlBasic/Counter  cnt_type=Free running  cnt_to=0  operation=Down  start_count=0  cnt_by_val=1  arith_type="Signed  (2's comp)"  n_bits=22  bin_pt=0  load_pin=on  rst=on  en=on  explicit_period=Explicit  period=FPGA_Ts  use_behavioral_HDL=off  implementation=DSP48  XmcBlockStatus=1  maskContainerNames=group1  block_type=counter  block_config=sysgen:Counter_config  block_width=531  block_height=1023
  inc_cntr1 : hdlBasic/Counter  cnt_type=Free running  cnt_to=0  operation=Down  start_count=0  cnt_by_val=1  arith_type="Signed  (2's comp)"  n_bits=22  bin_pt=0  load_pin=on  rst=on  en=on  explicit_period=Explicit  period=FPGA_Ts  use_behavioral_HDL=off  implementation=DSP48  XmcBlockStatus=1  maskContainerNames=group1  block_type=counter  block_config=sysgen:Counter_config  block_width=531  block_height=1023
  sign1 : hdlBasic/Slice  nbits=1  boolean_output=on  mode=Upper Bit Location + Width  bit1=0  base1=MSB of Input  bit0=0  base0=LSB of Input  XmcBlockStatus=1  maskContainerNames=group1  block_type=slice  block_config=sysgen:Slice_config
  upsample_hold_value : hdlBasic/Up Sample  sample_ratio=FPGA_CLK/PHCTRLR_CLK  copy_samples=on  en=off  latency=0  XmcBlockStatus=1  maskContainerNames=group1  block_type=usamp  block_config=sysgen:Upsample_config
  upsample_hold_value1 : hdlBasic/Up Sample  sample_ratio=FPGA_CLK/PHCTRLR_CLK  copy_samples=on  en=off  latency=0  XmcBlockStatus=1  maskContainerNames=group1  block_type=usamp  block_config=sysgen:Upsample_config
  INC_OUT : Outport
  DEC_OUT : Outport  Port=2
  read_clock_mon : Outport  Port=3
  wires:
  Logical14/1 -> Inverter/1
  Logical10/1 -> inc_cntr1/4
  Clock Enable Probe/1 -> Delay1/1
  Delay1/1 -> Logical1/1, Logical14/1, Logical10/1, inc_cntr1/1, inc_cntr/1, Logical11/1
  Inverter/1 -> Logical12/2
  Clock Enable Probe1/1 -> Logical13/1
  inc_cntr1/1 -> Relational1/1
  Logical7/1 -> Register/1
  upsample_hold_value1/1 -> Logical12/1
  Logical6/1 -> Logical7/2
  Logical11/1 -> inc_cntr/4
  Counter3/1 -> Relational3/1
  Logical8/1 -> Logical9/2
  puls_in/1 -> upsample_hold_value/1, Clock Enable Probe/1
  Constant2/1 -> Relational1/2
  Mux7/1 -> INC_OUT/1
  Constant5/1 -> Counter3/2
  reset/1 -> inc_cntr1/3, upsample_hold_value1/1
  Logical12/1 -> inc_cntr/3
  Constant6/1 -> Relational3/2
  Delay/1 -> Logical8/2
  Inverter3/1 -> Logical3/2
  Relational3/1 -> Mux1/1, Inverter3/1, Logical5/2  "counting"
  Relational5/1 -> Logical2/2, Mux8/3, Mux7/2
  Logical5/1 -> Counter3/3
  Register/1 -> Logical9/1, Logical7/1
  Inverter1/1 -> Logical6/2
  read_clk/1 -> Logical4/1, Mux1/2
  Logical9/1 -> Logical1/2, Logical2/1
  Logical4/1 -> Logical3/1
  Delay2/1 -> Mux1/3, Logical4/2
  Logical2/1 -> Logical11/2
  Absolute3/1 -> inc_cntr/2, inc_cntr1/2
  sign1/1 -> Mux8/1, Mux7/1
  Constant9/1 -> Relational5/2
  Logical13/1 -> Logical10/2
  Inverter4/1 -> Logical8/1
  Mux1/1 -> read_clock_mon/1, Delay2/1, Logical6/1, Inverter1/1, Inverter4/1, Delay/1
  Mux8/1 -> DEC_OUT/1
  Constant10/1 -> Mux8/2, Mux7/3
  Relational1/1 -> Logical14/2, Logical13/2
  Constant3/1 -> Clock Enable Probe1/1
  Logical3/1 -> Logical5/1, Counter3/1
  Logical1/1 -> Register/2
  inc_cntr/1 -> Relational5/1
  upsample_hold_value/1 -> sign1/1, Absolute3/1

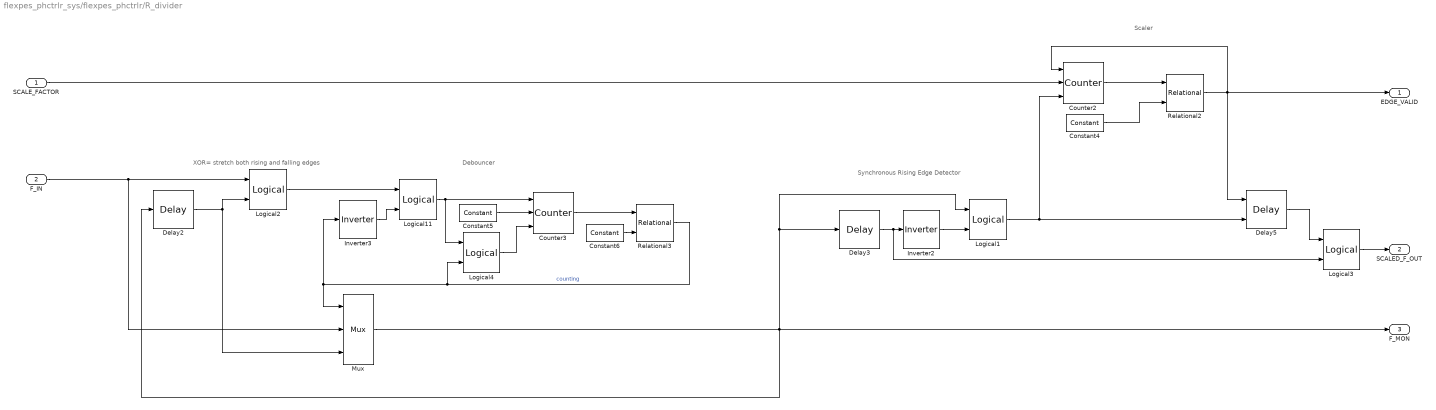
== system flexpes_phctrlr_sys/flexpes_phctrlr/R_divider ==
  note: XOR= stretch both rising and falling edges
  note: Debouncer
  note: Scaler
  note: Synchronous Rising Edge Detector
  SCALE_FACTOR : Inport
  F_IN : Inport  Port=2
  Constant4 : hdlBasic/Constant  const=1.0  gui_display_data_type=Fixed-point  arith_type=Unsigned  n_bits=16  bin_pt=0  preci_type=Single  exp_width=8  frac_width=24  explicit_period=off  period=1  XmcBlockStatus=1  maskContainerNames=tabcontainer1  block_type=constant  block_config=sysgen:Constant_config
  Constant5 : hdlBasic/Constant  const=debouncer_cycles  gui_display_data_type=Fixed-point  arith_type=Unsigned  n_bits=7  bin_pt=0  preci_type=Single  exp_width=8  frac_width=24  explicit_period=off  period=1  XmcBlockStatus=1  maskContainerNames=tabcontainer1  block_type=constant  block_config=sysgen:Constant_config
  Constant6 : hdlBasic/Constant  const=1  gui_display_data_type=Fixed-point  arith_type=Unsigned  n_bits=7  bin_pt=0  preci_type=Single  exp_width=8  frac_width=24  explicit_period=off  period=1  XmcBlockStatus=1  maskContainerNames=tabcontainer1  block_type=constant  block_config=sysgen:Constant_config
  Counter2 : hdlBasic/Counter  cnt_type=Free running  cnt_to=2  operation=Down  start_count=1  cnt_by_val=1  arith_type=Unsigned  n_bits=16  bin_pt=0  load_pin=on  rst=off  en=on  explicit_period=Explicit  period=FPGA_Ts  use_behavioral_HDL=off  implementation=Fabric  XmcBlockStatus=1  maskContainerNames=group1  block_type=counter  block_config=sysgen:Counter_config  block_width=531  block_height=1023
  Counter3 : hdlBasic/Counter  cnt_type=Free running  cnt_to=2  operation=Down  start_count=1  cnt_by_val=1  arith_type=Unsigned  n_bits=7  bin_pt=0  load_pin=on  rst=off  en=on  explicit_period=Explicit  period=FPGA_Ts  use_behavioral_HDL=off  implementation=Fabric  XmcBlockStatus=1  maskContainerNames=group1  block_type=counter  block_config=sysgen:Counter_config  block_width=531  block_height=1023
  Delay2 : hdlBasic/Delay  rst=off  en=off  latency=1  reg_retiming=off  XmcBlockStatus=1  maskContainerNames=group1  block_type=delay  block_config=sysgen:Delay_config
  Delay3 : hdlBasic/Delay  rst=off  en=off  latency=1  reg_retiming=off  XmcBlockStatus=1  maskContainerNames=group1  block_type=delay  block_config=sysgen:Delay_config
  Delay5 : hdlBasic/Delay  rst=off  en=on  latency=1  reg_retiming=off  XmcBlockStatus=1  maskContainerNames=group1  block_type=delay  block_config=sysgen:Delay_config
  Inverter2 : hdlBasic/Inverter  en=off  latency=0  XmcBlockStatus=1  maskContainerNames=group2  block_type=inv  block_config=sysgen:Inverter_config
  Inverter3 : hdlBasic/Inverter  en=off  latency=0  XmcBlockStatus=1  maskContainerNames=group2  block_type=inv  block_config=sysgen:Inverter_config
  Logical1 : hdlBasic/Logical  logical_function=AND  inputs=2  en=off  latency=0  precision=Full  arith_type=Unsigned  n_bits=16  bin_pt=0  align_bp=on  overflow=[]  quantization=[]  XmcBlockStatus=1  maskContainerNames=tabcontainer1  block_type=logical  block_config=sysgen:Logical_config
  Logical11 : hdlBasic/Logical  logical_function=AND  inputs=2  en=off  latency=0  precision=Full  arith_type=Unsigned  n_bits=16  bin_pt=0  align_bp=on  overflow=[]  quantization=[]  XmcBlockStatus=1  maskContainerNames=tabcontainer1  block_type=logical  block_config=sysgen:Logical_config
  Logical2 : hdlBasic/Logical  logical_function=XOR  inputs=2  en=off  latency=0  precision=Full  arith_type=Unsigned  n_bits=16  bin_pt=0  align_bp=on  overflow=[]  quantization=[]  XmcBlockStatus=1  maskContainerNames=tabcontainer1  block_type=logical  block_config=sysgen:Logical_config
  Logical3 : hdlBasic/Logical  logical_function=AND  inputs=2  en=off  latency=0  precision=Full  arith_type=Unsigned  n_bits=16  bin_pt=0  align_bp=on  overflow=[]  quantization=[]  XmcBlockStatus=1  maskContainerNames=tabcontainer1  block_type=logical  block_config=sysgen:Logical_config
  Logical4 : hdlBasic/Logical  logical_function=OR  inputs=2  en=off  latency=0  precision=Full  arith_type=Unsigned  n_bits=16  bin_pt=0  align_bp=on  overflow=[]  quantization=[]  XmcBlockStatus=1  maskContainerNames=tabcontainer1  block_type=logical  block_config=sysgen:Logical_config
  Mux : hdlBasic/Mux  inputs=2  en=off  latency=0  precision=Full  arith_type=Unsigned  n_bits=16  bin_pt=14  quantization=Truncate  overflow=Wrap  XmcBlockStatus=1  maskContainerNames=tabcontainer1  block_type=mux  block_config=sysgen:Mux_config
  Relational2 : hdlBasic/Relational  mode=a=b  op_type=Bool  en=off  latency=0  XmcBlockStatus=1  maskContainerNames=tabcontainer1  block_type=relational  block_config=sysgen:Relational_config
  Relational3 : hdlBasic/Relational  mode=a!=b  op_type=Bool  en=off  latency=0  XmcBlockStatus=1  maskContainerNames=tabcontainer1  block_type=relational  block_config=sysgen:Relational_config
  EDGE_VALID : Outport
  SCALED_F_OUT : Outport  Port=2
  F_MON : Outport  Port=3
  wires:
  Logical1/1 -> Counter2/3, Delay5/2
  Constant6/1 -> Relational3/2
  Inverter3/1 -> Logical11/2
  Counter3/1 -> Relational3/1
  Constant5/1 -> Counter3/2
  Relational3/1 -> Mux/1, Inverter3/1, Logical4/2  "counting"
  Delay5/1 -> Logical3/1
  Delay3/1 -> Inverter2/1, Logical3/2
  F_IN/1 -> Logical2/1, Mux/2
  Counter2/1 -> Relational2/1
  Inverter2/1 -> Logical1/2
  Constant4/1 -> Relational2/2
  SCALE_FACTOR/1 -> Counter2/2
  Logical11/1 -> Logical4/1, Counter3/1
  Logical3/1 -> SCALED_F_OUT/1
  Logical4/1 -> Counter3/3
  Logical2/1 -> Logical11/1
  Delay2/1 -> Mux/3, Logical2/2
  Relational2/1 -> EDGE_VALID/1, Delay5/1, Counter2/1
  Mux/1 -> F_MON/1, Delay2/1, Logical1/1, Delay3/1
